simulink model "XYSimulation"  (R2013b)
settings: Solver=ode45  StartTime=0.0  StopTime=13.71  RelTol=1e-3
values from neighbouring files (symbols this model uses):
  TrackWidth = 0.1    [parameters.m]
  WheelRadius = 0.035    [parameters.m]
libraries: simulink x1
settings Model: Creator=DEL  LastModifiedBy=DEL

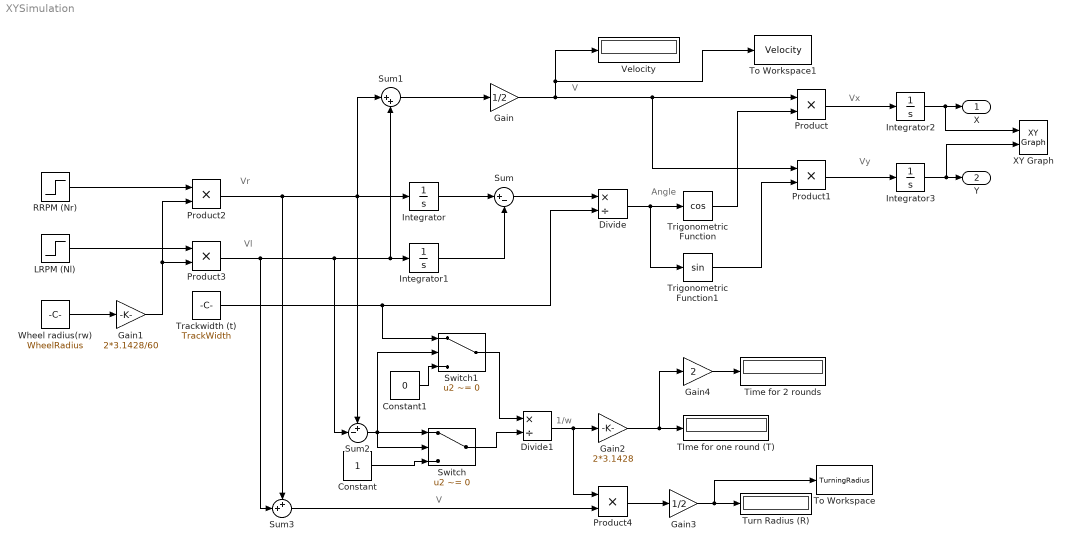
== system XYSimulation ==
  note: V
  note: 1/w
  note: Vl
  note: Vr
  note: Vy
  note: Vx
  note: Angle
  note: V
  Constant : Constant
  Constant1 : Constant  Value=0
  Divide : Product  Inputs=*/
  Divide1 : Product  Inputs=*/
  Gain : Gain  Gain=1/2
  Gain1 : Gain  Gain=2*3.1428/60
  Gain2 : Gain  Gain=2*3.1428
  Gain3 : Gain  Gain=1/2
  Gain4 : Gain  Gain=2
  Integrator{,1..3} (4 alike) : Integrator
  LRPM (Nl) : Step  Time=6.86  Before=120  After=145  SampleTime=0
  Product{,1..4} (5 alike) : Product
  RRPM (Nr) : Step  Time=6.86  Before=145  After=120  SampleTime=0
  Sum : Sum  Inputs=|+-
  Sum1 : Sum  Inputs=|++
  Sum2 : Sum  Inputs=+-|
  Sum3 : Sum  Inputs=++|
  Switch : Switch  Criteria=u2 ~= 0
  Switch1 : Switch  Criteria=u2 ~= 0
  TIme for one round (T) : Display
  Time for 2 rounds : Display
  To Workspace : ToWorkspace  VariableName=TurningRadius  SampleTime=-1
  To Workspace1 : ToWorkspace  VariableName=Velocity  SampleTime=-1
      settings: MaxDataPoints=1
  Trackwidth (t) : Constant  Value=TrackWidth
  Trigonometric Function : Trigonometry  Operator=cos
  Trigonometric Function1 : Trigonometry
  Turn Radius (R) : Display
  Velocity : Display
  Wheel radius(rw) : Constant  Value=WheelRadius
  XY Graph : simulink/Sinks/XY Graph  xmin=-1.2  xmax=1.2  ymin=-1.2  ymax=1.2  st=-1
  X : Outport
  Y : Outport  Port=2
  wires:
  Product3/1 -> Sum2/2, Sum1/2, Integrator1/1, Sum3/2
  Integrator/1 -> Sum/1
  Integrator1/1 -> Sum/2
  Sum/1 -> Divide/1
  Trackwidth (t)/1 -> Switch1/1, Divide/2
  Sum1/1 -> Gain/1
  Divide/1 -> Trigonometric Function/1, Trigonometric Function1/1
  Gain/1 -> Velocity/1, To Workspace1/1, Product/1, Product1/1
  Trigonometric Function/1 -> Product/2
  Trigonometric Function1/1 -> Product1/2
  Product/1 -> Integrator2/1
  Product1/1 -> Integrator3/1
  Integrator2/1 -> XY Graph/1, X/1
  Integrator3/1 -> XY Graph/2, Y/1
  RRPM (Nr)/1 -> Product2/1
  LRPM (Nl)/1 -> Product3/1
  Gain1/1 -> Product2/2, Product3/2
  Wheel radius(rw)/1 -> Gain1/1
  Gain2/1 -> Gain4/1, TIme for one round (T)/1
  Divide1/1 -> Product4/1, Gain2/1
  Product2/1 -> Integrator/1, Sum2/1, Sum1/1, Sum3/1
  Sum3/1 -> Product4/2
  Gain3/1 -> Turn Radius (R)/1, To Workspace/1
  Gain4/1 -> Time for 2 rounds/1
  Product4/1 -> Gain3/1
  Sum2/1 -> Switch1/2, Switch/1, Switch/2
  Switch/1 -> Divide1/2
  Constant/1 -> Switch/3
  Switch1/1 -> Divide1/1
  Constant1/1 -> Switch1/3
